simulink model "HRT20C"  (R2020a)
settings: Solver=ode23tb  StartTime=0  StopTime=2474  RelTol=1e-3  EnableMultiTasking=on
undefined symbols (not defined in the file): sigbuilder_block
libraries: autolibshared x2, simulink x1
(part 2 of 2)

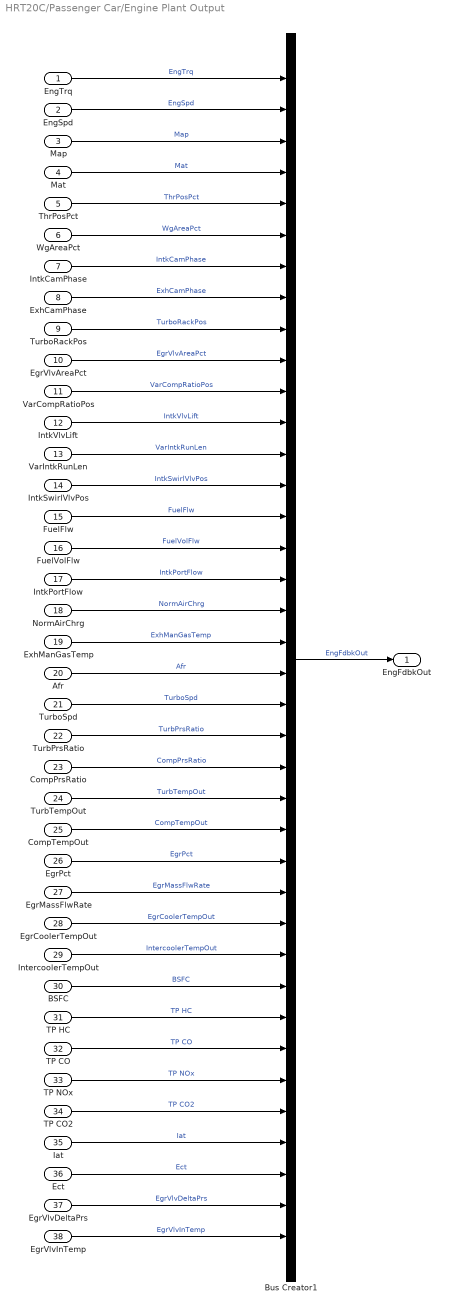
== system HRT20C/Passenger Car/Engine Plant Output ==
  EngTrq : Inport
  EngSpd : Inport  Port=2
  Map : Inport  Port=3
  Mat : Inport  Port=4
  ThrPosPct : Inport  Port=5
  WgAreaPct : Inport  Port=6
  IntkCamPhase : Inport  Port=7
  ExhCamPhase : Inport  Port=8
  TurboRackPos : Inport  Port=9
  EgrVlvAreaPct : Inport  Port=10
  VarCompRatioPos : Inport  Port=11
  IntkVlvLift : Inport  Port=12
  VarIntkRunLen : Inport  Port=13
  IntkSwirlVlvPos : Inport  Port=14
  FuelFlw : Inport  Port=15
  FuelVolFlw : Inport  Port=16
  IntkPortFlow : Inport  Port=17
  NormAirChrg : Inport  Port=18
  ExhManGasTemp : Inport  Port=19
  Afr : Inport  Port=20
  TurboSpd : Inport  Port=21
  TurbPrsRatio : Inport  Port=22
  CompPrsRatio : Inport  Port=23
  TurbTempOut : Inport  Port=24
  CompTempOut : Inport  Port=25
  EgrPct : Inport  Port=26
  EgrMassFlwRate : Inport  Port=27
  EgrCoolerTempOut : Inport  Port=28
  IntercoolerTempOut : Inport  Port=29
  BSFC : Inport  Port=30
  TP HC : Inport  Port=31
  TP CO : Inport  Port=32
  TP NOx : Inport  Port=33
  TP CO2 : Inport  Port=34
  Iat : Inport  Port=35
  Ect : Inport  Port=36
  EgrVlvDeltaPrs : Inport  Port=37
  EgrVlvInTemp : Inport  Port=38
  Bus Creator1 : BusCreator  Inputs=38
  EngFdbkOut : Outport  VectorParamsAs1DForOutWhenUnconnected=off
  wires:
  IntkSwirlVlvPos/1 -> Bus Creator1/14  "IntkSwirlVlvPos"
  VarIntkRunLen/1 -> Bus Creator1/13  "VarIntkRunLen"
  IntkVlvLift/1 -> Bus Creator1/12  "IntkVlvLift"
  VarCompRatioPos/1 -> Bus Creator1/11  "VarCompRatioPos"
  WgAreaPct/1 -> Bus Creator1/6  "WgAreaPct"
  TurboRackPos/1 -> Bus Creator1/9  "TurboRackPos"
  ThrPosPct/1 -> Bus Creator1/5  "ThrPosPct"
  EngTrq/1 -> Bus Creator1/1  "EngTrq"
  Mat/1 -> Bus Creator1/4  "Mat"
  Map/1 -> Bus Creator1/3  "Map"
  EngSpd/1 -> Bus Creator1/2  "EngSpd"
  IntkCamPhase/1 -> Bus Creator1/7  "IntkCamPhase"
  ExhCamPhase/1 -> Bus Creator1/8  "ExhCamPhase"
  EgrVlvAreaPct/1 -> Bus Creator1/10  "EgrVlvAreaPct"
  FuelFlw/1 -> Bus Creator1/15  "FuelFlw"
  IntkPortFlow/1 -> Bus Creator1/17  "IntkPortFlow"
  NormAirChrg/1 -> Bus Creator1/18  "NormAirChrg"
  ExhManGasTemp/1 -> Bus Creator1/19  "ExhManGasTemp"
  Afr/1 -> Bus Creator1/20  "Afr"
  TurboSpd/1 -> Bus Creator1/21  "TurboSpd"
  TurbPrsRatio/1 -> Bus Creator1/22  "TurbPrsRatio"
  CompPrsRatio/1 -> Bus Creator1/23  "CompPrsRatio"
  TurbTempOut/1 -> Bus Creator1/24  "TurbTempOut"
  CompTempOut/1 -> Bus Creator1/25  "CompTempOut"
  IntercoolerTempOut/1 -> Bus Creator1/29  "IntercoolerTempOut"
  EgrPct/1 -> Bus Creator1/26  "EgrPct"
  EgrMassFlwRate/1 -> Bus Creator1/27  "EgrMassFlwRate"
  EgrCoolerTempOut/1 -> Bus Creator1/28  "EgrCoolerTempOut"
  BSFC/1 -> Bus Creator1/30  "BSFC"
  TP HC/1 -> Bus Creator1/31  "TP HC"
  TP CO/1 -> Bus Creator1/32  "TP CO"
  TP NOx/1 -> Bus Creator1/33  "TP NOx"
  TP CO2/1 -> Bus Creator1/34  "TP CO2"
  Ect/1 -> Bus Creator1/36  "Ect"
  EgrVlvDeltaPrs/1 -> Bus Creator1/37  "EgrVlvDeltaPrs"
  EgrVlvInTemp/1 -> Bus Creator1/38  "EgrVlvInTemp"
  Iat/1 -> Bus Creator1/35  "Iat"
  Bus Creator1/1 -> EngFdbkOut/1  "EngFdbkOut"
  FuelVolFlw/1 -> Bus Creator1/16  "FuelVolFlw"

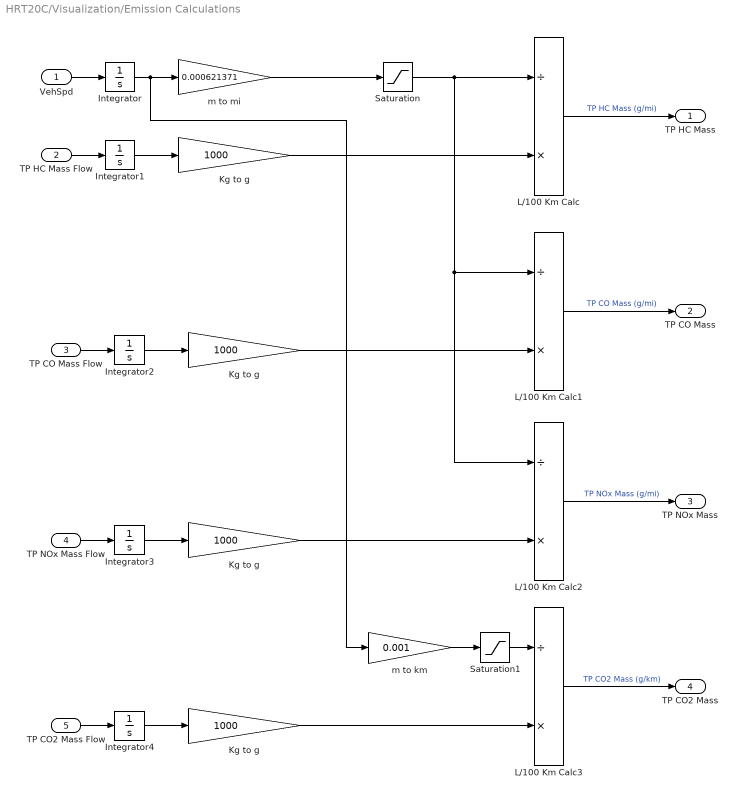
== system HRT20C/Visualization/Emission Calculations ==
  VehSpd : Inport
  TP HC Mass Flow : Inport  Port=2
  TP CO Mass Flow : Inport  Port=3
  TP NOx Mass Flow : Inport  Port=4
  TP CO2 Mass Flow : Inport  Port=5
  Integrator{,1..4} (5 alike) : Integrator
  Kg to g : Gain  Gain=1000
  "Kg to g " : Gain  Gain=1000
  "Kg to g  " : Gain  Gain=1000
  "Kg to g   " : Gain  Gain=1000
  L/100 Km Calc{,1..3} (4 alike) : Product  Inputs=/*
  Saturation : Saturate  UpperLimit=Inf  LowerLimit=0.2
  Saturation1 : Saturate  UpperLimit=Inf  LowerLimit=1
  m to km : Gain  Gain=0.001
  m to mi : Gain  Gain=0.000621371
  TP HC Mass : Outport  VectorParamsAs1DForOutWhenUnconnected=off
  TP CO Mass : Outport  Port=2  VectorParamsAs1DForOutWhenUnconnected=off
  TP NOx Mass : Outport  Port=3  VectorParamsAs1DForOutWhenUnconnected=off
  TP CO2 Mass : Outport  Port=4  VectorParamsAs1DForOutWhenUnconnected=off
  wires:
  L/100 Km Calc/1 -> TP HC Mass/1  "TP HC Mass (g/mi)"
  VehSpd/1 -> Integrator/1
  m to mi/1 -> Saturation/1
  Saturation/1 -> L/100 Km Calc2/1, L/100 Km Calc1/1, L/100 Km Calc/1
  TP HC Mass Flow/1 -> Integrator1/1
  Integrator1/1 -> Kg to g/1
  Integrator/1 -> m to km/1, m to mi/1
  Kg to g/1 -> L/100 Km Calc/2
  TP CO Mass Flow/1 -> Integrator2/1
  Integrator2/1 -> "Kg to g "/1
  "Kg to g "/1 -> L/100 Km Calc1/2
  TP NOx Mass Flow/1 -> Integrator3/1
  Integrator3/1 -> "Kg to g  "/1
  "Kg to g  "/1 -> L/100 Km Calc2/2
  L/100 Km Calc1/1 -> TP CO Mass/1  "TP CO Mass (g/mi)"
  L/100 Km Calc2/1 -> TP NOx Mass/1  "TP NOx Mass (g/mi)"
  TP CO2 Mass Flow/1 -> Integrator4/1
  Integrator4/1 -> "Kg to g   "/1
  "Kg to g   "/1 -> L/100 Km Calc3/2
  L/100 Km Calc3/1 -> TP CO2 Mass/1  "TP CO2 Mass (g/km)"
  Saturation1/1 -> L/100 Km Calc3/1
  m to km/1 -> Saturation1/1

== system HRT20C/Visualization/Performance Calculations ==
  VehSpd : Inport
  FuelVolFlow : Inport  Port=2
  Integrator : Integrator
  Integrator1 : Integrator
  L/100 Km Calc : Product  Inputs=/*
  Product : Product
  Saturation : Saturate  UpperLimit=Inf  LowerLimit=0.001
  Saturation1 : Saturate  UpperLimit=Inf  LowerLimit=1e-3
  Sqrt : Sqrt  SaturateOnIntegerOverflow=on
  US MPG Calc : Product  Inputs=*/
  m to 100Km : Gain  Gain=1/1000/100
  m to mile : Gain  Gain=0.000621371
  m^3 to L : Gain  Gain=1000
  m^3 to US Gal : Gain  Gain=264.172
  US MPG : Outport  VectorParamsAs1DForOutWhenUnconnected=off
  L/100Km : Outport  Port=2  VectorParamsAs1DForOutWhenUnconnected=off
  wires:
  m^3 to US Gal/1 -> Saturation1/1
  m^3 to L/1 -> L/100 Km Calc/2
  Integrator/1 -> m to mile/1, m to 100Km/1
  m to mile/1 -> US MPG Calc/1
  FuelVolFlow/1 -> Integrator1/1
  Integrator1/1 -> m^3 to US Gal/1, m^3 to L/1
  Saturation/1 -> L/100 Km Calc/1
  m to 100Km/1 -> Saturation/1
  VehSpd/1 -> Product/2, Product/1
  L/100 Km Calc/1 -> L/100Km/1  "L/100Km"
  US MPG Calc/1 -> US MPG/1  "US MPG"
  Saturation1/1 -> US MPG Calc/2
  Product/1 -> Sqrt/1
  Sqrt/1 -> Integrator/1

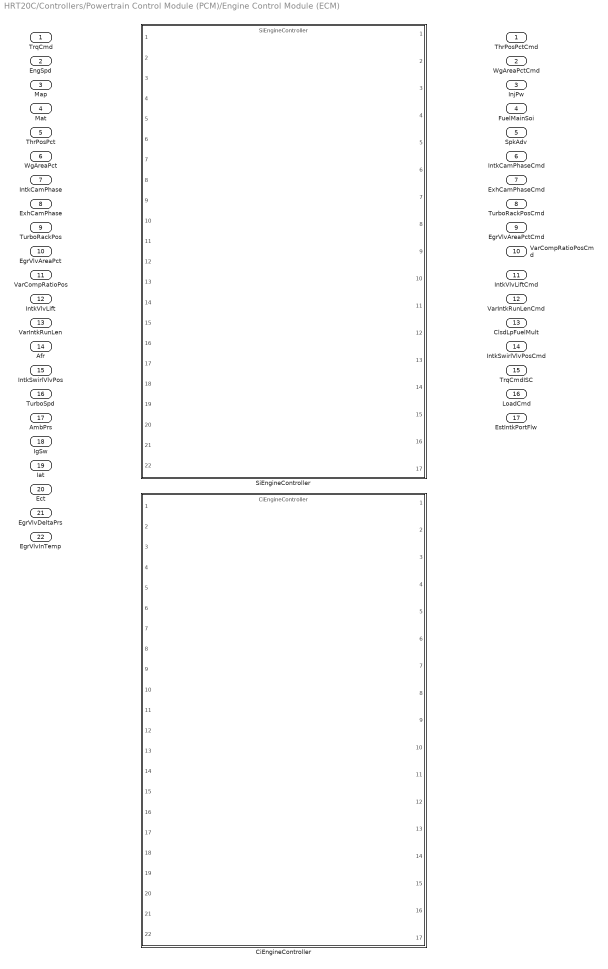
== system HRT20C/Controllers/Powertrain Control Module (PCM)/Engine Control Module (ECM) ==
  TrqCmd : Inport
  EngSpd : Inport  Port=2
  Map : Inport  Port=3
  Mat : Inport  Port=4
  ThrPosPct : Inport  Port=5
  WgAreaPct : Inport  Port=6
  IntkCamPhase : Inport  Port=7
  ExhCamPhase : Inport  Port=8
  TurboRackPos : Inport  Port=9
  EgrVlvAreaPct : Inport  Port=10
  VarCompRatioPos : Inport  Port=11
  IntkVlvLift : Inport  Port=12
  VarIntkRunLen : Inport  Port=13
  Afr : Inport  Port=14
  IntkSwirlVlvPos : Inport  Port=15
  TurboSpd : Inport  Port=16
  AmbPrs : Inport  Port=17
  IgSw : Inport  Port=18
  Iat : Inport  Port=19
  Ect : Inport  Port=20
  EgrVlvDeltaPrs : Inport  Port=21
  EgrVlvInTemp : Inport  Port=22
  CiEngineController : ModelReference  ModelNameDialog=CiEngineController.slx  SimulationMode=Normal  VariantControl=CiEngineController  ModelReferenceVersion=1.243
  SiEngineController : ModelReference  ModelNameDialog=SiEngineController.slx  SimulationMode=Normal  VariantControl=SiEngineController  ModelReferenceVersion=1.306
  ThrPosPctCmd : Outport  VectorParamsAs1DForOutWhenUnconnected=off
  WgAreaPctCmd : Outport  Port=2  VectorParamsAs1DForOutWhenUnconnected=off
  InjPw : Outport  Port=3  VectorParamsAs1DForOutWhenUnconnected=off
  FuelMainSoi : Outport  Port=4  VectorParamsAs1DForOutWhenUnconnected=off
  SpkAdv : Outport  Port=5  VectorParamsAs1DForOutWhenUnconnected=off
  IntkCamPhaseCmd : Outport  Port=6  VectorParamsAs1DForOutWhenUnconnected=off
  ExhCamPhaseCmd : Outport  Port=7  VectorParamsAs1DForOutWhenUnconnected=off
  TurboRackPosCmd : Outport  Port=8  VectorParamsAs1DForOutWhenUnconnected=off
  EgrVlvAreaPctCmd : Outport  Port=9  VectorParamsAs1DForOutWhenUnconnected=off
  VarCompRatioPosCmd : Outport  Port=10  VectorParamsAs1DForOutWhenUnconnected=off
  IntkVlvLiftCmd : Outport  Port=11  VectorParamsAs1DForOutWhenUnconnected=off
  VarIntkRunLenCmd : Outport  Port=12  VectorParamsAs1DForOutWhenUnconnected=off
  ClsdLpFuelMult : Outport  Port=13  VectorParamsAs1DForOutWhenUnconnected=off
  IntkSwirlVlvPosCmd : Outport  Port=14  VectorParamsAs1DForOutWhenUnconnected=off
  TrqCmdISC : Outport  Port=15  VectorParamsAs1DForOutWhenUnconnected=off
  LoadCmd : Outport  Port=16  VectorParamsAs1DForOutWhenUnconnected=off
  EstIntkPortFlw : Outport  Port=17  VectorParamsAs1DForOutWhenUnconnected=off

== system HRT20C/Controllers/Powertrain Control Module (PCM)/Powertrain Torque Structure Control ==
  AccCmd : Inport
  DecCmd : Inport  Port=2
  Acc to Torque Request : Gain  Gain=180
  Brake Pressure Command : Gain  Gain=8e6
  Unit Delay : UnitDelay  SampleTime=0.01  HasFrameUpgradeWarning=on
  BrakeCmd : Outport  VectorParamsAs1DForOutWhenUnconnected=off
  EngTrqReq : Outport  Port=2  VectorParamsAs1DForOutWhenUnconnected=off
  wires:
  Acc to Torque Request/1 -> EngTrqReq/1  "EngineTrqReq"
  DecCmd/1 -> Unit Delay/1
  AccCmd/1 -> Acc to Torque Request/1
  Unit Delay/1 -> Brake Pressure Command/1
  Brake Pressure Command/1 -> BrakeCmd/1

== system HRT20C/Controllers/Powertrain Control Module (PCM)/Transmission Control Module (TCM) ==
  AccCmd : Inport
  VehSpdFdbk : Inport  Port=2
  EngSpdFdbk : Inport  Port=3
  PowertrainBestFuelController : ModelReference  ModelNameDialog=PowertrainBestFuelController.slx  SimulationMode=Normal  VariantControl=PowertrainBestFuelController  ModelReferenceVersion=1.196
  PowertrainMaxPowerController : ModelReference  ModelNameDialog=PowertrainMaxPowerController.slx  SimulationMode=Normal  VariantControl=PowertrainMaxPowerController  ModelReferenceVersion=1.149
  TransmissionCmd : Outport  VectorParamsAs1DForOutWhenUnconnected=off

== system HRT20C/Longitudinal Driver/Longitudinal Driver/Enabled Subsystem ==
  xdot : Inport
  Enable : EnablePort
  100 KPH Performance Test Threshold : simulink/Logic and Bit Operations/Compare To Constant  relop=>=  const=100  OutDataTypeStr=boolean
  m/s to kph : Gain  Gain=3.6
  100 KPH Reached : Outport  VectorParamsAs1DForOutWhenUnconnected=off
  wires:
  100 KPH Performance Test Threshold/1 -> 100 KPH Reached/1
  xdot/1 -> m/s to kph/1
  m/s to kph/1 -> 100 KPH Performance Test Threshold/1

== system HRT20C/Longitudinal Driver/Longitudinal Driver/Ignition Switch Profile ==
  Demux : Demux  Tag=STV Demux  Outputs=1
      settings: DisplayOption=none
  FromWs : FromWorkspace  Tag=STV FromWs  VariableName=tuvar
      SigBuilderData=|
      | common.afterFinalStr = 'Extrapolate'
      | common.sampleTime = 0
      | dataSet.timeRange = [0 10]
      | dataSet.name = 'Group 1'
      | sbobj.Groups.Name = 'Group 1'
      | sbobj.Groups.Signals.Name = 'IGSW'
      | sbobj.Groups.Signals.XData = [0 5 5 6 6 10]
      | sbobj.Groups.Signals.YData = [0 0 1 1 0 0]
  IGSW : Outport  Tag=STV Outport  VectorParamsAs1DForOutWhenUnconnected=off
  wires:
  FromWs/1 -> Demux/1
  Demux/1 -> IGSW/1

== system HRT20C/Longitudinal Driver/Longitudinal Driver/W.O.T. ==
  EngSpd : Inport
  DriverInfo : Inport  Port=2
  Bus Assignment : BusAssignment  AssignedSignals=Accel
  Slip Limited Acc : Lookup_n-D  NumberOfTableDimensions=1  BreakpointsForDimension1=[5000 6000]  Table=[1 0]  ExtrapMethod=Clip  InternalRulePriority=Speed  RndMeth=Simplest  InputSameDT=on
  Acc : Outport  VectorParamsAs1DForOutWhenUnconnected=off
  wires:
  EngSpd/1 -> Slip Limited Acc/1
  Slip Limited Acc/1 -> Bus Assignment/2  "Accel"
  Bus Assignment/1 -> Acc/1  "Info"
  DriverInfo/1 -> Bus Assignment/1

== system HRT20C/Longitudinal Driver/Open Loop/Ignition Switch Profile ==
  Demux : Demux  Tag=STV Demux  Outputs=1
      settings: DisplayOption=none
  FromWs : FromWorkspace  Tag=STV FromWs  VariableName=tuvar
      SigBuilderData=|
      | common.afterFinalStr = 'Extrapolate'
      | common.sampleTime = 0
      | dataSet.timeRange = [0 10]
      | dataSet.name = 'Group 1'
      | sbobj.Groups.Name = 'Group 1'
      | sbobj.Groups.Signals.Name = 'IGSW'
      | sbobj.Groups.Signals.XData = [0 5 5 6 6 10]
      | sbobj.Groups.Signals.YData = [0 0 1 1 0 0]
  IGSW : Outport  Tag=STV Outport  VectorParamsAs1DForOutWhenUnconnected=off
  wires:
  Demux/1 -> IGSW/1
  FromWs/1 -> Demux/1
